simulink model "communication_Arduino"  (R2023b)
settings: Solver=VariableStepAuto  StartTime=0.0  StopTime=1  FixedStep=0.001  RelTol=1e-3  AbsTol=1e-3
undefined symbols (not defined in the file): g, LF, robot_conversions, robot_joints, X, Y, Z
libraries: sm_lib x13, nesl_utility x7, simulink_extras x6, cstblocks x6, instrumentseriallib x3, simulink x3
settings Model: Creator=ivano  LastModifiedBy=ivano
settings SolverCC: AlgebraicLoopSolver=TrustRegion  MaxZcPerStep=1
settings DataIOCC: LimitDataPoints=on  MaxDataPoints=10000  ReturnWorkspaceOutputs=off  ReturnWorkspaceOutputsName=data
settings OptimizationCC: DefaultParameterBehavior=Inlined  EnhancedBackFolding=on  PassReuseOutputArgsAs=Individual arguments  ZeroExternalMemoryAtStartup=off  ZeroInternalMemoryAtStartup=off  MaxStackSize=64  OptimizeBlockOrder=speed  DifferentSizesBufferReuse=on  OptimizationCustomize=off  EfficientTunableParamExpr=on
settings DebuggingCC: ParameterTunabilityLossMsg=error  UnconnectedInputMsg=warning  UnconnectedOutputMsg=warning  UnconnectedLineMsg=warning  AllowSymbolicDim=off  SubsystemReferenceDiagnosticForUnitTest=warning  SFUnexpectedBacktrackingDiag=warning  SFNoUnconditionalDefaultTransitionDiag=warning  SFExecutionAtInitializationDiag=none  ArithmeticOperatorsInVariantConditions=warning
settings HardwareCC: ProdBitPerPointer=32  ProdBitPerSizeT=32  ProdBitPerPtrDiffT=32  ProdLargestAtomicInteger=Long  ProdLargestAtomicFloat=Double  ProdWordSize=32  ProdHWDeviceType=ARM Compatible->ARM Cortex
settings ModelReferenceCC: EnableRefExpFcnMdlSchedulingChecks=on
settings SFSimCC: SimUseLocalCustomCode=off  MATLABDynamicMemAlloc=off  CustomCodeUndefinedFunction=UseInterfaceOnly  SimTargetLang=C++  GPUAcceleration=on  SimDLTargetLibrary=cudnn
settings RTWCC: Description=Embedded Coder  SystemTargetFile=ert.tlc  TemplateMakefile=ert_default_tmf  RTWUseLocalCustomCode=off  BuildConfiguration=Faster Runs  DLArmComputeVersion=19.05
settings CodeAppCC: ForceParamTrailComments=on  IgnoreCustomStorageClasses=off  OperatorAnnotations=on  SimulinkDataObjDesc=on  SFDataObjDesc=on  InsertBlockDesc=on
settings ERTTargetCC: SupportContinuousTime=on  ExtModeTransport=3  ExtModeStaticAlloc=on  ExtModeStaticAllocSize=24576  ExtModeMexFile=ext_xcp  ExtModeIntrfLevel=Level2 - Open  ERTCustomFileTemplate=example_file_process.tlc
settings ConfigComp: CovMetricSettings=dw  CovSaveCumulativeToWorkspaceVar=on  CovSaveSingleToWorkspaceVar=on  CovExternalEMLEnable=off  CovSFcnEnable=off
settings SimscapeCC: SimscapeLogType=all  SimscapeLogSimulationStatistics=on  SimscapeLogDataHistory=10000

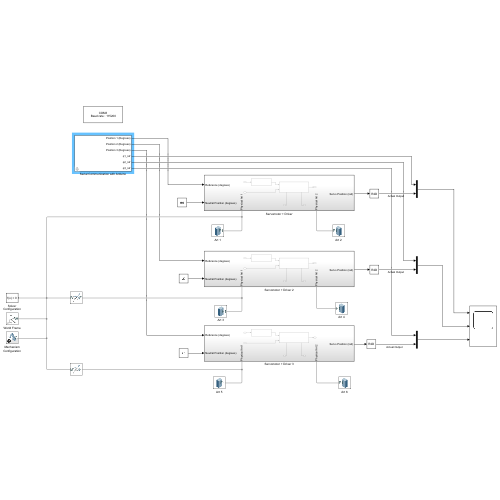
[thumbnail: Simulink's stored preview of the top-level diagram]
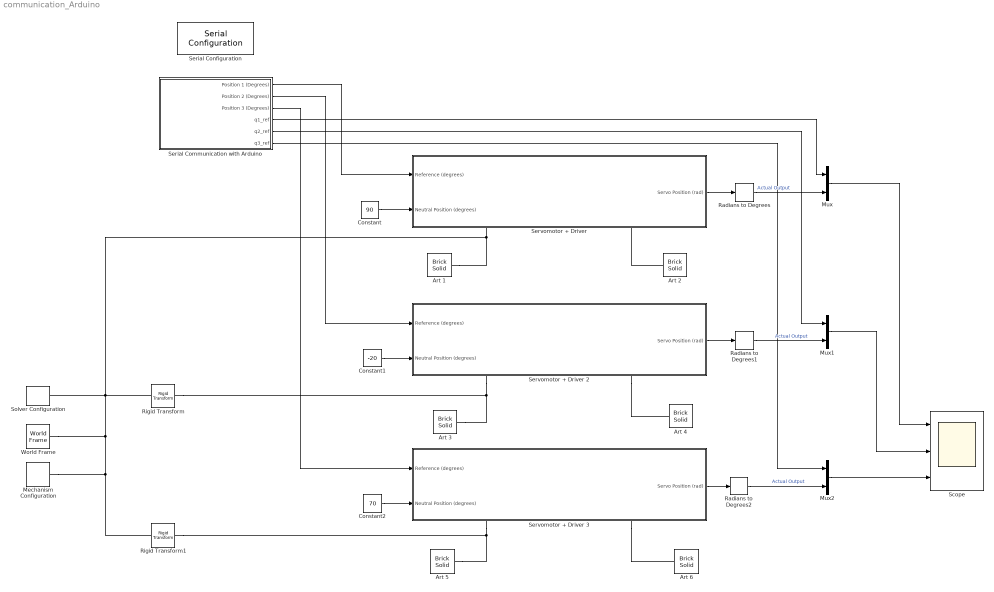
== system communication_Arduino ==
  Art 1 : sm_lib/Body Elements/Brick Solid  GraphicAmbientColor=[0.15 0.15 0.15 1.0]  BasedOnType=Density  BrickDimensions=[1 1 1]  BrickDimensionsUnits=m  CenterOfMass=[0 0 0]  CenterOfMassUnits=m  GraphicDiffuseColor=[0.0 0.8 0.8]  Density=10  DensityUnits=kg/m^3  DoExposeReferenceFrame=off  GraphicEmissiveColor=[0.0 0.0 0.0 1.0]  ExportEntireGeometry=off  SerializedFrames=<Frames><Frame><Id>Frame1</Id><Value><Name>F1</Name><Origin><Source>GeometricFeature</Source><FeatureName>+z surface</FeatureName></Origin><PrimaryAxis><DefinedDirection>+Z</DefinedDirection><Source>ReferenceFrame</Source><SourceDirection>+Z</SourceDirection><FeatureName></FeatureName></PrimaryAxis><SecondaryAxis><DefinedDirection>+X</DefinedDirection><Source>ReferenceFrame</Source><SourceDirection>+X</SourceDirection><FeatureName></FeatureName></SecondaryAxis></Value></Frame></Frames>  MarkerShape=Sphere  MarkerSize=10  GraphicType=FromGeometry  InertiaType=CalculateFromGeometry  Mass=1  MassUnits=kg  MomentsOfInertia=[1 1 1]  MomentsOfInertiaUnits=kg*m^2  GraphicOpacity=1.0  ProductsOfInertia=[0 0 0]  ProductsOfInertiaUnits=kg*m^2  GraphicShininess=75  GraphicSpecularColor=[0.5 0.5 0.5 1.0]  GraphicVisPropType=SimpleVisualProperties
  Art 2 : sm_lib/Body Elements/Brick Solid  GraphicAmbientColor=[0.15 0.15 0.15 1.0]  BasedOnType=Density  BrickDimensions=[3 1 1]  BrickDimensionsUnits=m  CenterOfMass=[0 0 0]  CenterOfMassUnits=m  GraphicDiffuseColor=[0.8 0.8 1.0]  Density=10  DensityUnits=kg/m^3  DoExposeReferenceFrame=off  GraphicEmissiveColor=[0.0 0.0 0.0 1.0]  ExportEntireGeometry=off  SerializedFrames=<Frames><Frame><Id>Frame1</Id><Value><Name>F1</Name><Origin><Source>GeometricFeature</Source><FeatureName>+z surface</FeatureName></Origin><PrimaryAxis><DefinedDirection>-Z</DefinedDirection><Source>ReferenceFrame</Source><SourceDirection>+Z</SourceDirection><FeatureName></FeatureName></PrimaryAxis><SecondaryAxis><DefinedDirection>+X</DefinedDirection><Source>ReferenceFrame</Source><SourceDirection>+X</SourceDirection><FeatureName></FeatureName></SecondaryAxis></Value></Frame></Frames>  MarkerShape=Sphere  MarkerSize=10  GraphicType=FromGeometry  InertiaType=CalculateFromGeometry  Mass=1  MassUnits=kg  MomentsOfInertia=[1 1 1]  MomentsOfInertiaUnits=kg*m^2  GraphicOpacity=1.0  ProductsOfInertia=[0 0 0]  ProductsOfInertiaUnits=kg*m^2  GraphicShininess=75  GraphicSpecularColor=[0.5 0.5 0.5 1.0]  GraphicVisPropType=SimpleVisualProperties
  Art 3 : sm_lib/Body Elements/Brick Solid  GraphicAmbientColor=[0.15 0.15 0.15 1.0]  BasedOnType=Density  BrickDimensions=[1 1 1]  BrickDimensionsUnits=m  CenterOfMass=[0 0 0]  CenterOfMassUnits=m  GraphicDiffuseColor=[0.0 0.8 0.8]  Density=10  DensityUnits=kg/m^3  DoExposeReferenceFrame=off  GraphicEmissiveColor=[0.0 0.0 0.0 1.0]  ExportEntireGeometry=off  SerializedFrames=<Frames><Frame><Id>Frame1</Id><Value><Name>F1</Name><Origin><Source>GeometricFeature</Source><FeatureName>+z surface</FeatureName></Origin><PrimaryAxis><DefinedDirection>+Z</DefinedDirection><Source>ReferenceFrame</Source><SourceDirection>+Z</SourceDirection><FeatureName></FeatureName></PrimaryAxis><SecondaryAxis><DefinedDirection>+X</DefinedDirection><Source>ReferenceFrame</Source><SourceDirection>+X</SourceDirection><FeatureName></FeatureName></SecondaryAxis></Value></Frame></Frames>  MarkerShape=Sphere  MarkerSize=10  GraphicType=FromGeometry  InertiaType=CalculateFromGeometry  Mass=1  MassUnits=kg  MomentsOfInertia=[1 1 1]  MomentsOfInertiaUnits=kg*m^2  GraphicOpacity=1.0  ProductsOfInertia=[0 0 0]  ProductsOfInertiaUnits=kg*m^2  GraphicShininess=75  GraphicSpecularColor=[0.5 0.5 0.5 1.0]  GraphicVisPropType=SimpleVisualProperties
  Art 4 : sm_lib/Body Elements/Brick Solid  GraphicAmbientColor=[0.15 0.15 0.15 1.0]  BasedOnType=Density  BrickDimensions=[3 1 1]  BrickDimensionsUnits=m  CenterOfMass=[0 0 0]  CenterOfMassUnits=m  GraphicDiffuseColor=[0.8 0.8 1.0]  Density=10  DensityUnits=kg/m^3  DoExposeReferenceFrame=off  GraphicEmissiveColor=[0.0 0.0 0.0 1.0]  ExportEntireGeometry=off  SerializedFrames=<Frames><Frame><Id>Frame1</Id><Value><Name>F1</Name><Origin><Source>GeometricFeature</Source><FeatureName>+z surface</FeatureName></Origin><PrimaryAxis><DefinedDirection>-Z</DefinedDirection><Source>ReferenceFrame</Source><SourceDirection>+Z</SourceDirection><FeatureName></FeatureName></PrimaryAxis><SecondaryAxis><DefinedDirection>+X</DefinedDirection><Source>ReferenceFrame</Source><SourceDirection>+X</SourceDirection><FeatureName></FeatureName></SecondaryAxis></Value></Frame></Frames>  MarkerShape=Sphere  MarkerSize=10  GraphicType=FromGeometry  InertiaType=CalculateFromGeometry  Mass=1  MassUnits=kg  MomentsOfInertia=[1 1 1]  MomentsOfInertiaUnits=kg*m^2  GraphicOpacity=1.0  ProductsOfInertia=[0 0 0]  ProductsOfInertiaUnits=kg*m^2  GraphicShininess=75  GraphicSpecularColor=[0.5 0.5 0.5 1.0]  GraphicVisPropType=SimpleVisualProperties
  Art 5 : sm_lib/Body Elements/Brick Solid  GraphicAmbientColor=[0.15 0.15 0.15 1.0]  BasedOnType=Density  BrickDimensions=[1 1 1]  BrickDimensionsUnits=m  CenterOfMass=[0 0 0]  CenterOfMassUnits=m  GraphicDiffuseColor=[0.0 0.8 0.8]  Density=10  DensityUnits=kg/m^3  DoExposeReferenceFrame=off  GraphicEmissiveColor=[0.0 0.0 0.0 1.0]  ExportEntireGeometry=off  SerializedFrames=<Frames><Frame><Id>Frame1</Id><Value><Name>F1</Name><Origin><Source>GeometricFeature</Source><FeatureName>+z surface</FeatureName></Origin><PrimaryAxis><DefinedDirection>+Z</DefinedDirection><Source>ReferenceFrame</Source><SourceDirection>+Z</SourceDirection><FeatureName></FeatureName></PrimaryAxis><SecondaryAxis><DefinedDirection>+X</DefinedDirection><Source>ReferenceFrame</Source><SourceDirection>+X</SourceDirection><FeatureName></FeatureName></SecondaryAxis></Value></Frame></Frames>  MarkerShape=Sphere  MarkerSize=10  GraphicType=FromGeometry  InertiaType=CalculateFromGeometry  Mass=1  MassUnits=kg  MomentsOfInertia=[1 1 1]  MomentsOfInertiaUnits=kg*m^2  GraphicOpacity=1.0  ProductsOfInertia=[0 0 0]  ProductsOfInertiaUnits=kg*m^2  GraphicShininess=75  GraphicSpecularColor=[0.5 0.5 0.5 1.0]  GraphicVisPropType=SimpleVisualProperties
  Art 6 : sm_lib/Body Elements/Brick Solid  GraphicAmbientColor=[0.15 0.15 0.15 1.0]  BasedOnType=Density  BrickDimensions=[3 1 1]  BrickDimensionsUnits=m  CenterOfMass=[0 0 0]  CenterOfMassUnits=m  GraphicDiffuseColor=[0.8 0.8 1.0]  Density=10  DensityUnits=kg/m^3  DoExposeReferenceFrame=off  GraphicEmissiveColor=[0.0 0.0 0.0 1.0]  ExportEntireGeometry=off  SerializedFrames=<Frames><Frame><Id>Frame1</Id><Value><Name>F1</Name><Origin><Source>GeometricFeature</Source><FeatureName>+z surface</FeatureName></Origin><PrimaryAxis><DefinedDirection>-Z</DefinedDirection><Source>ReferenceFrame</Source><SourceDirection>+Z</SourceDirection><FeatureName></FeatureName></PrimaryAxis><SecondaryAxis><DefinedDirection>+X</DefinedDirection><Source>ReferenceFrame</Source><SourceDirection>+X</SourceDirection><FeatureName></FeatureName></SecondaryAxis></Value></Frame></Frames>  MarkerShape=Sphere  MarkerSize=10  GraphicType=FromGeometry  InertiaType=CalculateFromGeometry  Mass=1  MassUnits=kg  MomentsOfInertia=[1 1 1]  MomentsOfInertiaUnits=kg*m^2  GraphicOpacity=1.0  ProductsOfInertia=[0 0 0]  ProductsOfInertiaUnits=kg*m^2  GraphicShininess=75  GraphicSpecularColor=[0.5 0.5 0.5 1.0]  GraphicVisPropType=SimpleVisualProperties
  Constant : Constant  Value=90
  Constant1 : Constant  Value=-20
  Constant2 : Constant  Value=70
  Mechanism Configuration : sm_lib/Utilities/Mechanism Configuration  UniformGravity=Constant  GravityVector=[0 0 g]  GravityVectorUnits=m/s^2  LinearizationDelta=0.001  JointModeTransitionNonlinearIterations=2
  Mux : Mux  Inputs=2
  Mux1 : Mux  Inputs=2
  Mux2 : Mux  Inputs=2
  Radians to Degrees : simulink_extras/Transformations/Radians to Degrees
  Radians to Degrees1 : simulink_extras/Transformations/Radians to Degrees
  Radians to Degrees2 : simulink_extras/Transformations/Radians to Degrees
  Rigid Transform : sm_lib/Frames and Transforms/Rigid Transform  TranslationMethod=Cartesian  TranslationStandardOffset=0  TranslationStandardOffsetUnits=m  TranslationStandardAxis=+Z  TranslationCartesianOffset=[5 0 0]  TranslationCartesianOffsetUnits=m  TranslationROffset=0  TranslationROffsetUnits=m  TranslationZOffset=0  TranslationZOffsetUnits=m  TranslationThetaOffset=0  TranslationThetaOffsetUnits=deg  RotationMethod=None  RotationAngleUnits=deg  RotationStandardAxis=+Z  RotationAngle=0.0  RotationArbitraryAxis=[0 0 1]  FollAlignAxisA=+X  BaseAlignAxisA=+Y  FollAlignAxisB=+Y  BaseAlignAxisB=+Z  RotationSequenceAxes=FollowerAxes  RotationSequence=XYX  RotationSequenceAngles=[0 0 0]  RotationSequenceAnglesUnits=deg  RotationMatrix=[1 0 0; 0 1 0; 0 0 1]  Quaternion=[1 0 0 0]
  Rigid Transform1 : sm_lib/Frames and Transforms/Rigid Transform  TranslationMethod=Cartesian  TranslationStandardOffset=0  TranslationStandardOffsetUnits=m  TranslationStandardAxis=+Z  TranslationCartesianOffset=[0 5 0]  TranslationCartesianOffsetUnits=m  TranslationROffset=0  TranslationROffsetUnits=m  TranslationZOffset=0  TranslationZOffsetUnits=m  TranslationThetaOffset=0  TranslationThetaOffsetUnits=deg  RotationMethod=None  RotationAngleUnits=deg  RotationStandardAxis=+Z  RotationAngle=0.0  RotationArbitraryAxis=[0 0 1]  FollAlignAxisA=+X  BaseAlignAxisA=+Y  FollAlignAxisB=+Y  BaseAlignAxisB=+Z  RotationSequenceAxes=FollowerAxes  RotationSequence=XYX  RotationSequenceAngles=[0 0 0]  RotationSequenceAnglesUnits=deg  RotationMatrix=[1 0 0; 0 1 0; 0 0 1]  Quaternion=[1 0 0 0]
  Scope : Scope  NumInputPorts=3
  Serial Communication with Arduino : Subsystem  mask{q1=0, q2=0, q3=0}
  Serial Configuration : instrumentseriallib/Serial Configuration  Priority=-200000  PortSel=COM3  Port=COM3  ComPort=COM3  BaudRate=115200  DataBits=8  Parity=none  StopBits=1  ByteOrder=little-endian  FlowControl=none  Timeout=10  SimulateUsing=Interpreted execution  BlockInModel=on  aMode=1
  Servomotor + Driver : Subsystem
      settings: PortSchema="{\"entries\":[{\"content\":{\"sides\":[{\"content\":{\"connectorIds\":[\"In1\",\"In2\"]},\"type\":\"ConnectorPlacement.EquallySpacedRectSide\",\"uuid\":\"34aed934-2639-4a00-aaee-cf3027466446\"},{\"content\":{\"connectorIds\":[\"Out1\"],\"side\":\"RIGHT\"},\"type\":\"ConnectorPlacement.EquallySpacedRectSide\",\"uuid\":\"6801890d-3466-4e37-90e8-6d1471e5b2c4\"},{\"content\":{\"side\":\"TOP\"},\"type\":\"ConnectorPlacement.EquallySpacedRectSide\",\"uuid\":\"bc3191aa-eca4-4e32-9fcf-8d5b7059b0b6\"},{\"content\":{\"connectorIds\":[\"RConn1\",\"RConn2\"],\"side\":\"BOTTOM\"},\"type\":\"ConnectorPlacement.EquallySpacedRectSide\",\"uuid\":\"867f09f9-bc2c-4353-bf05-5e7fc6d76fc7\"}]},\"type\":\"ConnectorPlacement.EquallySpacedConnector\",\"uuid\":\"7616468a-464c-41b8-bfd7-188201b948eb\"}],\"packageUris\":[\"http://schema.mathworks.com/mf0/Connector/R2020b\"],\"version\":\"1.0\"}"
  Servomotor + Driver 2 : Subsystem
      settings: PortSchema="{\"entries\":[{\"content\":{\"sides\":[{\"content\":{\"connectorIds\":[\"In1\",\"In2\"]},\"type\":\"ConnectorPlacement.EquallySpacedRectSide\",\"uuid\":\"34aed934-2639-4a00-aaee-cf3027466446\"},{\"content\":{\"connectorIds\":[\"Out1\"],\"side\":\"RIGHT\"},\"type\":\"ConnectorPlacement.EquallySpacedRectSide\",\"uuid\":\"6801890d-3466-4e37-90e8-6d1471e5b2c4\"},{\"content\":{\"side\":\"TOP\"},\"type\":\"ConnectorPlacement.EquallySpacedRectSide\",\"uuid\":\"bc3191aa-eca4-4e32-9fcf-8d5b7059b0b6\"},{\"content\":{\"connectorIds\":[\"RConn1\",\"RConn2\"],\"side\":\"BOTTOM\"},\"type\":\"ConnectorPlacement.EquallySpacedRectSide\",\"uuid\":\"867f09f9-bc2c-4353-bf05-5e7fc6d76fc7\"}]},\"type\":\"ConnectorPlacement.EquallySpacedConnector\",\"uuid\":\"7616468a-464c-41b8-bfd7-188201b948eb\"}],\"packageUris\":[\"http://schema.mathworks.com/mf0/Connector/R2020b\"],\"version\":\"1.0\"}"
  Servomotor + Driver 3 : Subsystem
      settings: PortSchema="{\"entries\":[{\"content\":{\"sides\":[{\"content\":{\"connectorIds\":[\"In1\",\"In2\"]},\"type\":\"ConnectorPlacement.EquallySpacedRectSide\",\"uuid\":\"34aed934-2639-4a00-aaee-cf3027466446\"},{\"content\":{\"connectorIds\":[\"Out1\"],\"side\":\"RIGHT\"},\"type\":\"ConnectorPlacement.EquallySpacedRectSide\",\"uuid\":\"6801890d-3466-4e37-90e8-6d1471e5b2c4\"},{\"content\":{\"side\":\"TOP\"},\"type\":\"ConnectorPlacement.EquallySpacedRectSide\",\"uuid\":\"bc3191aa-eca4-4e32-9fcf-8d5b7059b0b6\"},{\"content\":{\"connectorIds\":[\"RConn1\",\"RConn2\"],\"side\":\"BOTTOM\"},\"type\":\"ConnectorPlacement.EquallySpacedRectSide\",\"uuid\":\"867f09f9-bc2c-4353-bf05-5e7fc6d76fc7\"}]},\"type\":\"ConnectorPlacement.EquallySpacedConnector\",\"uuid\":\"7616468a-464c-41b8-bfd7-188201b948eb\"}],\"packageUris\":[\"http://schema.mathworks.com/mf0/Connector/R2020b\"],\"version\":\"1.0\"}"
  Solver Configuration : nesl_utility/Solver Configuration  PhysicalDomain=network_engine_domain  SubClassName=solver  LeftPortType=input  RightPortType=generic  Tones=[]  Harmonics=[]  SimulateNoise=off  Profile=off  UseLocalSampling=off  EnableSwitchedLinearOptims=on  FrequencyDomain=off  UseCCode=off  RelTol=0.001  AbsTol=1e-06  MinStep=1e-09  ToWorkspace=off  RevertToSquareIcSolve=off  NumHomotopyIterations=100  PhasorMode=off  PhasorModeNumHarmonics=1  ConsistencySolver=NEWTON_XTOL_AFTER_FTOL  IndexReductionMethod=DerivativeReplacement  DoDC=off  ResidualTolerance=1e-09  ConsistencyTolSource=GLOBAL  ConsistencyAbsTol=0.001  ConsistencyRelTol=0.001  ConsistencyTolFactor=0.001  UseLocalSolver=off  LocalSolverChoice=NE_BACKWARD_EULER_ADVANCER  ResolveIndetEquations=on  FunctionEvalNumThread=1  LocalSolverSampleTime=0.001  DoFixedCost=off  MaxNonlinIter=3  MaxModeIter=2  ComputeImpulses=off  ImpulseIterations=2  LinearAlgebra=Sparse  LinearAlgebraNumThread=0  EquationFormulation=NE_TIME_EF  DelaysMemoryBudget=1024  AutomaticFiltering=on  FilteringTimeConstant=0.001  PartitionStorageMethod=AS_NEEDED  PartitionMemoryBudget=1024  PartitionMethod=FAST  MultibodyUseLocalSolver=off  MultibodyLocalSolverChoice=ODE1  MultibodyLocalSolverSampleTime=0.001
  World Frame : sm_lib/Frames and Transforms/World Frame
  wires:
  Radians to Degrees/1 -> Mux/2  "Actual Output"
  Mux/1 -> Scope/1
  Servomotor + Driver/1(Servo Position (rad)) -> Radians to Degrees/1
  Radians to Degrees1/1 -> Mux1/2  "Actual Output"
  Mux1/1 -> Scope/2
  Servomotor + Driver 2/1(Servo Position (rad)) -> Radians to Degrees1/1
  Radians to Degrees2/1 -> Mux2/2  "Actual Output"
  Mux2/1 -> Scope/3
  Servomotor + Driver 3/1(Servo Position (rad)) -> Radians to Degrees2/1
  Serial Communication with Arduino/4(q1_ref) -> Mux/1
  Serial Communication with Arduino/5(q2_ref) -> Mux1/1
  Serial Communication with Arduino/6(q3_ref) -> Mux2/1
  Serial Communication with Arduino/1(Position 1 (Degrees)) -> Servomotor + Driver/1(Reference (degrees))
  Serial Communication with Arduino/2(Position 2 (Degrees)) -> Servomotor + Driver 2/1(Reference (degrees))
  Serial Communication with Arduino/3(Position 3 (Degrees)) -> Servomotor + Driver 3/1(Reference (degrees))
  Constant/1 -> Servomotor + Driver/2(Neutral Position (degrees))
  Constant1/1 -> Servomotor + Driver 2/2(Neutral Position (degrees))
  Constant2/1 -> Servomotor + Driver 3/2(Neutral Position (degrees))
  connections:
  World Frame/RConn1 -- Rigid Transform/LConn1 -- Art 1/LConn1 -- Servomotor + Driver/RConn1 -- Solver Configuration/RConn1 -- Mechanism Configuration/RConn1 -- Rigid Transform1/LConn1
  Art 2/LConn1 -- Servomotor + Driver/RConn2
  Art 3/LConn1 -- Servomotor + Driver 2/RConn1 -- Rigid Transform/RConn1
  Servomotor + Driver 2/RConn2 -- Art 4/LConn1
  Art 5/LConn1 -- Servomotor + Driver 3/RConn1 -- Rigid Transform1/RConn1
  Servomotor + Driver 3/RConn2 -- Art 6/LConn1

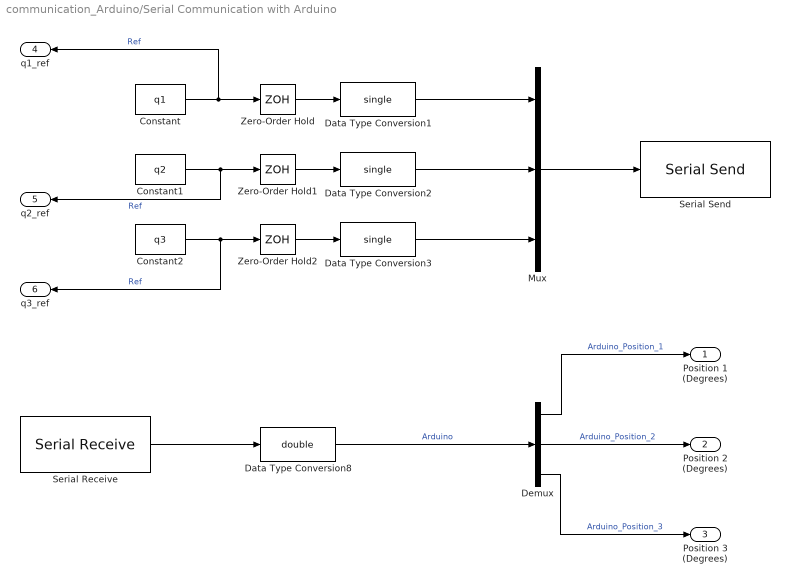
== system communication_Arduino/Serial Communication with Arduino ==
  Constant : Constant  Value=q1
  Constant1 : Constant  Value=q2
  Constant2 : Constant  Value=q3
  Data Type Conversion1 : DataTypeConversion  OutDataTypeStr=single  SaturateOnIntegerOverflow=off  RndMeth=Floor
  Data Type Conversion2 : DataTypeConversion  OutDataTypeStr=single  SaturateOnIntegerOverflow=off  RndMeth=Floor
  Data Type Conversion3 : DataTypeConversion  OutDataTypeStr=single  SaturateOnIntegerOverflow=off  RndMeth=Floor
  Data Type Conversion8 : DataTypeConversion  OutDataTypeStr=double  SaturateOnIntegerOverflow=off  RndMeth=Floor
  Demux : Demux  Outputs=3
  Mux : Mux  Inputs=3
  Serial Receive : instrumentseriallib/Serial Receive  Priority=1  PortSel=COM3  Port=COM3  ComPort=COM3  DataType=single  SaveDataType=uint8  ToggleHeader=on  Header='S'  DataSize=[3 1]  ToggleTerminator=on  Terminator=LF ('\n')  CustomTerminator=[]  InputFormat=Column major  ToggleDataSize=on  EnableBlockingMode=on  ActionDataUnavailable=Output last received value  ActionWhenDataUnavailable=Output last received value  CustomValue=0  SampleTime=0.01  SimulateUsing=Interpreted execution  BlockInModel=on  aMode=1
  Serial Send : instrumentseriallib/Serial Send  Priority=1  PortSel=COM3  Port=COM3  ComPort=COM3  Header='A'  Terminator=LF ('\n')  CustomTerminator=[]  EnableBlockingMode=on  SimulateUsing=Interpreted execution  BlockInModel=on  aMode=1
  Zero-Order Hold : ZeroOrderHold  SampleTime=0.01
  Zero-Order Hold1 : ZeroOrderHold  SampleTime=0.01
  Zero-Order Hold2 : ZeroOrderHold  SampleTime=0.01
  Position 1 (Degrees) : Outport
  Position 2 (Degrees) : Outport  Port=2
  Position 3 (Degrees) : Outport  Port=3
  q1_ref : Outport  Port=4
  q2_ref : Outport  Port=5
  q3_ref : Outport  Port=6
  wires:
  Constant/1 -> q1_ref/1, Zero-Order Hold/1  "Ref"
  Zero-Order Hold/1 -> Data Type Conversion1/1
  Constant1/1 -> q2_ref/1, Zero-Order Hold1/1  "Ref"
  Zero-Order Hold1/1 -> Data Type Conversion2/1
  Constant2/1 -> q3_ref/1, Zero-Order Hold2/1  "Ref"
  Zero-Order Hold2/1 -> Data Type Conversion3/1
  Data Type Conversion1/1 -> Mux/1
  Data Type Conversion2/1 -> Mux/2
  Data Type Conversion3/1 -> Mux/3
  Mux/1 -> Serial Send/1
  Demux/1 -> Position 1 (Degrees)/1  "Arduino_Position_1"
  Demux/2 -> Position 2 (Degrees)/1  "Arduino_Position_2"
  Demux/3 -> Position 3 (Degrees)/1  "Arduino_Position_3"
  Serial Receive/1 -> Data Type Conversion8/1
  Data Type Conversion8/1 -> Demux/1  "Arduino"

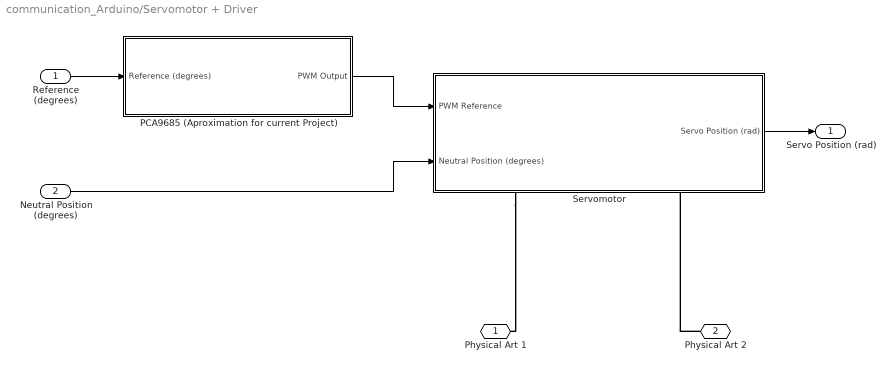
== system communication_Arduino/Servomotor + Driver ==
  Reference (degrees) : Inport
  Neutral Position (degrees) : Inport  Port=2
  PCA9685 (Aproximation for current Project) : Subsystem
  Servomotor : Subsystem
      settings: PortSchema="{\"entries\":[{\"content\":{\"sides\":[{\"content\":{\"connectorIds\":[\"In1\",\"In2\"]},\"type\":\"ConnectorPlacement.EquallySpacedRectSide\",\"uuid\":\"eeff66d3-7cb0-4fe9-90b5-92935711e170\"},{\"content\":{\"connectorIds\":[\"Out1\"],\"side\":\"RIGHT\"},\"type\":\"ConnectorPlacement.EquallySpacedRectSide\",\"uuid\":\"4c1729b3-3224-4ed4-9eed-359312bd5e7e\"},{\"content\":{\"side\":\"TOP\"},\"type\":\"ConnectorPlacement.EquallySpacedRectSide\",\"uuid\":\"ee6ed6e9-0c82-482d-bf53-5898b89012ab\"},{\"content\":{\"connectorIds\":[\"RConn1\",\"RConn2\"],\"side\":\"BOTTOM\"},\"type\":\"ConnectorPlacement.EquallySpacedRectSide\",\"uuid\":\"6da00c0c-ced6-4450-8de1-d587d7c692e9\"}]},\"type\":\"ConnectorPlacement.EquallySpacedConnector\",\"uuid\":\"38b9234f-cec7-4245-8a78-4426dc0791bf\"}],\"packageUris\":[\"http://schema.mathworks.com/mf0/Connector/R2020b\"],\"version\":\"1.0\"}"
  Physical Art 1 : PMIOPort  Side=Right
  Physical Art 2 : PMIOPort  Port=2  Side=Right
  Servo Position (rad) : Outport
  wires:
  PCA9685 (Aproximation for current Project)/1(PWM Output) -> Servomotor/1(PWM Reference)
  Neutral Position (degrees)/1 -> Servomotor/2(Neutral Position (degrees))
  Reference (degrees)/1 -> PCA9685 (Aproximation for current Project)/1(Reference (degrees))
  Servomotor/1(Servo Position (rad)) -> Servo Position (rad)/1
  connections:
  Servomotor/RConn1 -- Physical Art 1/RConn1
  Physical Art 2/RConn1 -- Servomotor/RConn2

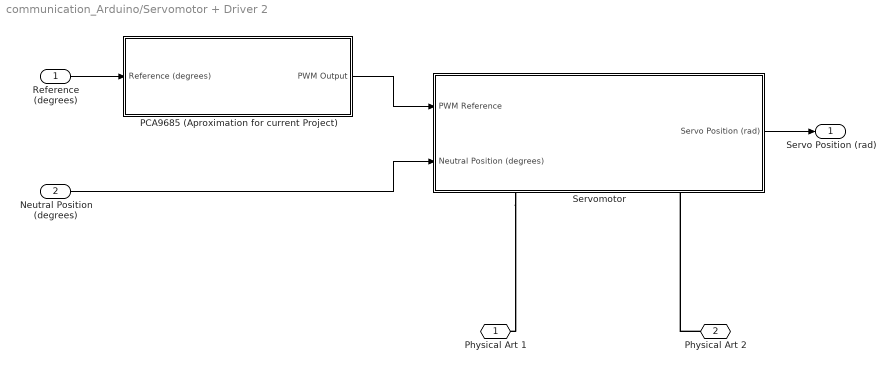
== system communication_Arduino/Servomotor + Driver 2 ==
  Reference (degrees) : Inport
  Neutral Position (degrees) : Inport  Port=2
  PCA9685 (Aproximation for current Project) : Subsystem
  Servomotor : Subsystem
      settings: PortSchema="{\"entries\":[{\"content\":{\"sides\":[{\"content\":{\"connectorIds\":[\"In1\",\"In2\"]},\"type\":\"ConnectorPlacement.EquallySpacedRectSide\",\"uuid\":\"eeff66d3-7cb0-4fe9-90b5-92935711e170\"},{\"content\":{\"connectorIds\":[\"Out1\"],\"side\":\"RIGHT\"},\"type\":\"ConnectorPlacement.EquallySpacedRectSide\",\"uuid\":\"4c1729b3-3224-4ed4-9eed-359312bd5e7e\"},{\"content\":{\"side\":\"TOP\"},\"type\":\"ConnectorPlacement.EquallySpacedRectSide\",\"uuid\":\"ee6ed6e9-0c82-482d-bf53-5898b89012ab\"},{\"content\":{\"connectorIds\":[\"RConn1\",\"RConn2\"],\"side\":\"BOTTOM\"},\"type\":\"ConnectorPlacement.EquallySpacedRectSide\",\"uuid\":\"6da00c0c-ced6-4450-8de1-d587d7c692e9\"}]},\"type\":\"ConnectorPlacement.EquallySpacedConnector\",\"uuid\":\"38b9234f-cec7-4245-8a78-4426dc0791bf\"}],\"packageUris\":[\"http://schema.mathworks.com/mf0/Connector/R2020b\"],\"version\":\"1.0\"}"
  Physical Art 1 : PMIOPort  Side=Right
  Physical Art 2 : PMIOPort  Port=2  Side=Right
  Servo Position (rad) : Outport
  wires:
  PCA9685 (Aproximation for current Project)/1(PWM Output) -> Servomotor/1(PWM Reference)
  Neutral Position (degrees)/1 -> Servomotor/2(Neutral Position (degrees))
  Reference (degrees)/1 -> PCA9685 (Aproximation for current Project)/1(Reference (degrees))
  Servomotor/1(Servo Position (rad)) -> Servo Position (rad)/1
  connections:
  Servomotor/RConn1 -- Physical Art 1/RConn1
  Physical Art 2/RConn1 -- Servomotor/RConn2

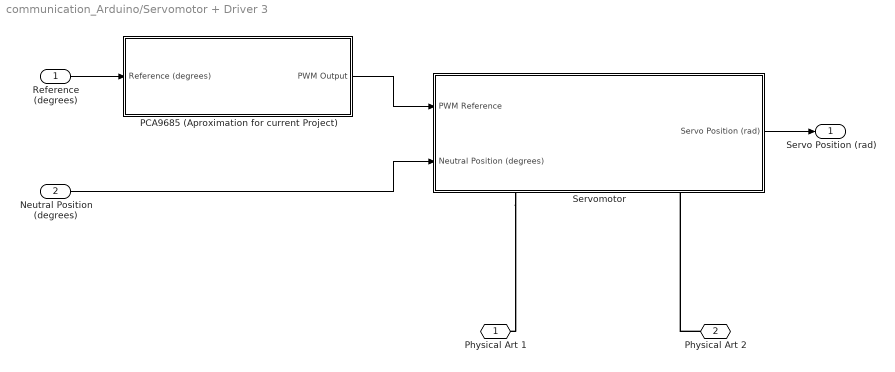
== system communication_Arduino/Servomotor + Driver 3 ==
  Reference (degrees) : Inport
  Neutral Position (degrees) : Inport  Port=2
  PCA9685 (Aproximation for current Project) : Subsystem
  Servomotor : Subsystem
      settings: PortSchema="{\"entries\":[{\"content\":{\"sides\":[{\"content\":{\"connectorIds\":[\"In1\",\"In2\"]},\"type\":\"ConnectorPlacement.EquallySpacedRectSide\",\"uuid\":\"eeff66d3-7cb0-4fe9-90b5-92935711e170\"},{\"content\":{\"connectorIds\":[\"Out1\"],\"side\":\"RIGHT\"},\"type\":\"ConnectorPlacement.EquallySpacedRectSide\",\"uuid\":\"4c1729b3-3224-4ed4-9eed-359312bd5e7e\"},{\"content\":{\"side\":\"TOP\"},\"type\":\"ConnectorPlacement.EquallySpacedRectSide\",\"uuid\":\"ee6ed6e9-0c82-482d-bf53-5898b89012ab\"},{\"content\":{\"connectorIds\":[\"RConn1\",\"RConn2\"],\"side\":\"BOTTOM\"},\"type\":\"ConnectorPlacement.EquallySpacedRectSide\",\"uuid\":\"6da00c0c-ced6-4450-8de1-d587d7c692e9\"}]},\"type\":\"ConnectorPlacement.EquallySpacedConnector\",\"uuid\":\"38b9234f-cec7-4245-8a78-4426dc0791bf\"}],\"packageUris\":[\"http://schema.mathworks.com/mf0/Connector/R2020b\"],\"version\":\"1.0\"}"
  Physical Art 1 : PMIOPort  Side=Right
  Physical Art 2 : PMIOPort  Port=2  Side=Right
  Servo Position (rad) : Outport
  wires:
  PCA9685 (Aproximation for current Project)/1(PWM Output) -> Servomotor/1(PWM Reference)
  Neutral Position (degrees)/1 -> Servomotor/2(Neutral Position (degrees))
  Reference (degrees)/1 -> PCA9685 (Aproximation for current Project)/1(Reference (degrees))
  Servomotor/1(Servo Position (rad)) -> Servo Position (rad)/1
  connections:
  Servomotor/RConn1 -- Physical Art 1/RConn1
  Physical Art 2/RConn1 -- Servomotor/RConn2

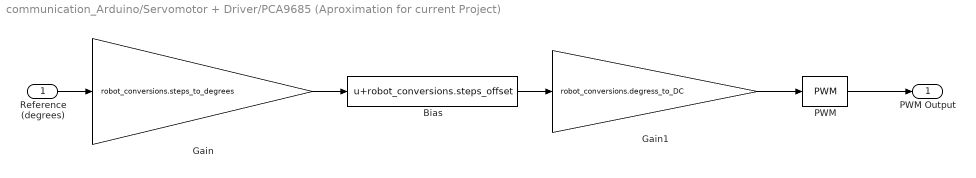
== system communication_Arduino/Servomotor + Driver/PCA9685 (Aproximation for current Project) ==
  Reference (degrees) : Inport
  Bias : Bias  Bias=robot_conversions.steps_offset  SaturateOnIntegerOverflow=off
  Gain : Gain  Gain=robot_conversions.steps_to_degrees
  Gain1 : Gain  Gain=robot_conversions.degress_to_DC
  PWM : simulink/Discontinuities/PWM  DisableCoverage=on  Period=0.02  InitialDelay=0  DisallowZeroDutyCycle=off  RunAtFixedTimeIntervals=off  SampleTime=0.01
  PWM Output : Outport
  wires:
  Gain/1 -> Bias/1
  Bias/1 -> Gain1/1
  Gain1/1 -> PWM/1
  Reference (degrees)/1 -> Gain/1
  PWM/1 -> PWM Output/1

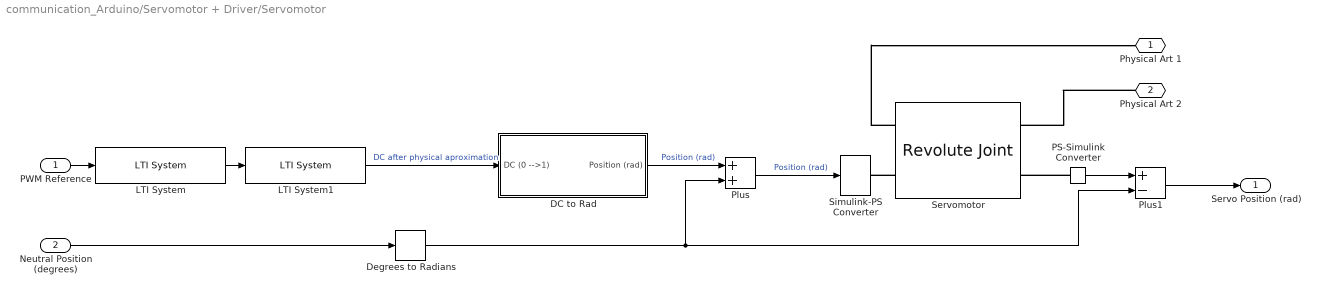
== system communication_Arduino/Servomotor + Driver/Servomotor ==
  PWM Reference : Inport
  Neutral Position (degrees) : Inport  Port=2
  DC to Rad : Subsystem
  Degrees to Radians : simulink_extras/Transformations/Degrees to Radians
  LTI System : cstblocks/LTI System  sys=robot_tf.bessel_filter  IC=[]  PadeOrder=0
  LTI System1 : cstblocks/LTI System  sys=robot_tf.physical_tf  IC=[]  PadeOrder=0
  PS-Simulink Converter : nesl_utility/PS-Simulink Converter  PhysicalDomain=network_engine_domain  SubClassName=ps_output  LeftPortType=input  RightPortType=output  PseudoPeriodic=off  Frequencies=[]  VectorFormat=inherit  Unit=inherit  AffineConversion=off
  Plus : Sum
  Plus1 : Sum  Inputs=+-
  Servomotor : sm_lib/Joints/Revolute Joint  JointMode=Normal  SenseConstraintForce=off  SenseConstraintForceX=off  SenseConstraintForceY=off  SenseConstraintForceZ=off  SenseConstraintTorque=off  SenseConstraintTorqueX=off  SenseConstraintTorqueY=off  SenseConstraintTorqueZ=off  SenseTotalForce=off  SenseTotalForceX=off  SenseTotalForceY=off  SenseTotalForceZ=off  SenseTotalTorque=off  SenseTotalTorqueX=off  SenseTotalTorqueY=off  SenseTotalTorqueZ=off  CompositeWrenchDir=FollowerOnBase  CompositeWrenchFrame=BaseFrame  EquilibriumPosition=0  EquilibriumPositionUnits=rad  SpringStiffness=0  SpringStiffnessUnits=N*m/deg  DampingCoefficient=0  DampingCoefficientUnits=N*m/(deg/s)  TorqueActuationMode=ComputedTorque  MotionActuationMode=InputMotion  SensePosition=on  SenseVelocity=off  SenseAcceleration=off  SenseTorqueForce=off  SenseLowerLimitTorqueForce=off  SenseUpperLimitTorqueForce=off  LowerLimitSpecify=on  LowerLimitBound=robot_joints.q_limits(1)  LowerLimitBoundUnits=rad  LowerLimitStiffness=1e4  LowerLimitStiffnessUnits=N*m/deg  LowerLimitDamping=10  LowerLimitDampingUnits=N*m/(deg/s)  LowerLimitTransitionRegionWidth=0.1  LowerLimitTransitionRegionWidthUnits=deg  UpperLimitSpecify=on  UpperLimitBound=robot_joints.q_limits(2)  UpperLimitBoundUnits=rad  UpperLimitStiffness=1e4  UpperLimitStiffnessUnits=N*m/deg  UpperLimitDamping=10  UpperLimitDampingUnits=N*m/(deg/s)  UpperLimitTransitionRegionWidth=0.1  UpperLimitTransitionRegionWidthUnits=deg  PositionTargetSpecify=off  PositionTargetPriority=High  PositionTargetValue=0  PositionTargetValueUnits=deg  VelocityTargetSpecify=off  VelocityTargetPriority=High  VelocityTargetValue=0  VelocityTargetValueUnits=deg/s
  Simulink-PS Converter : nesl_utility/Simulink-PS Converter  PhysicalDomain=network_engine_domain  SubClassName=ps_input  LeftPortType=input  RightPortType=output  PseudoPeriodic=off  Frequencies=[]  NoiseDistribution=none  NoiseParameters=[]  Unit=1  AffineConversion=off  FilteringAndDerivatives=filter  SimscapeFilterOrder=2  InputFilterTimeConstant=0.001  UdotUserProvided=0
  Physical Art 1 : PMIOPort  Side=Right
  Physical Art 2 : PMIOPort  Port=2  Side=Right
  Servo Position (rad) : Outport
  wires:
  PWM Reference/1 -> LTI System/1
  LTI System/1 -> LTI System1/1
  LTI System1/1 -> DC to Rad/1(DC (0 -->1))  "DC after physical aproximation"
  Neutral Position (degrees)/1 -> Degrees to Radians/1
  DC to Rad/1(Position (rad)) -> Plus/1  "Position (rad)"
  Plus/1 -> Simulink-PS Converter/1  "Position (rad)"
  Degrees to Radians/1 -> Plus1/2, Plus/2
  PS-Simulink Converter/1 -> Plus1/1
  Plus1/1 -> Servo Position (rad)/1
  connections:
  PS-Simulink Converter/LConn1 -- Servomotor/RConn2
  Physical Art 2/RConn1 -- Servomotor/RConn1
  Servomotor/LConn1 -- Physical Art 1/RConn1
  Servomotor/LConn2 -- Simulink-PS Converter/RConn1

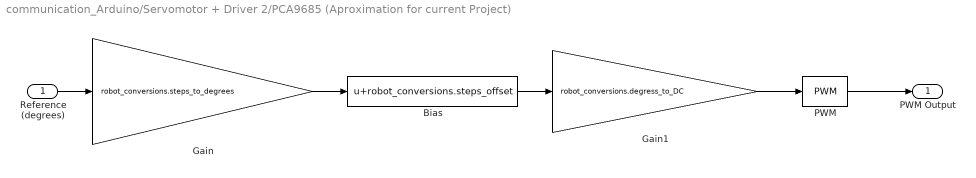
== system communication_Arduino/Servomotor + Driver 2/PCA9685 (Aproximation for current Project) ==
  Reference (degrees) : Inport
  Bias : Bias  Bias=robot_conversions.steps_offset  SaturateOnIntegerOverflow=off
  Gain : Gain  Gain=robot_conversions.steps_to_degrees
  Gain1 : Gain  Gain=robot_conversions.degress_to_DC
  PWM : simulink/Discontinuities/PWM  DisableCoverage=on  Period=0.02  InitialDelay=0  DisallowZeroDutyCycle=off  RunAtFixedTimeIntervals=off  SampleTime=0.01
  PWM Output : Outport
  wires:
  Gain/1 -> Bias/1
  Bias/1 -> Gain1/1
  Gain1/1 -> PWM/1
  Reference (degrees)/1 -> Gain/1
  PWM/1 -> PWM Output/1

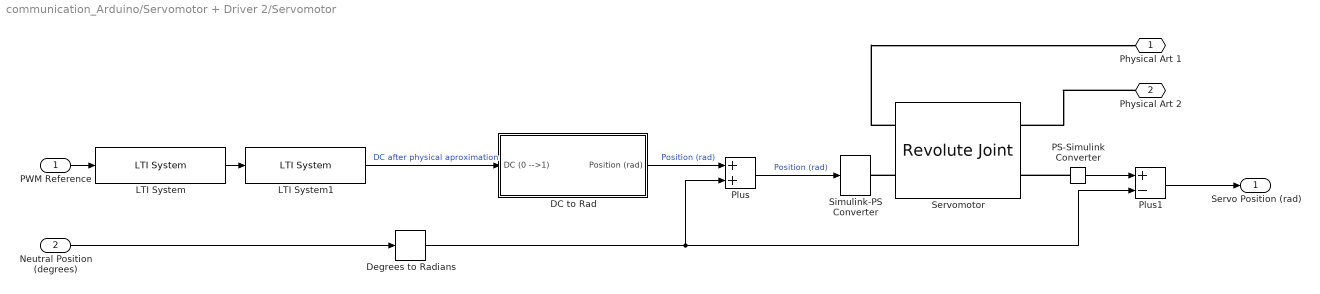
== system communication_Arduino/Servomotor + Driver 2/Servomotor ==
  PWM Reference : Inport
  Neutral Position (degrees) : Inport  Port=2
  DC to Rad : Subsystem
  Degrees to Radians : simulink_extras/Transformations/Degrees to Radians
  LTI System : cstblocks/LTI System  sys=robot_tf.bessel_filter  IC=[]  PadeOrder=0
  LTI System1 : cstblocks/LTI System  sys=robot_tf.physical_tf  IC=[]  PadeOrder=0
  PS-Simulink Converter : nesl_utility/PS-Simulink Converter  PhysicalDomain=network_engine_domain  SubClassName=ps_output  LeftPortType=input  RightPortType=output  PseudoPeriodic=off  Frequencies=[]  VectorFormat=inherit  Unit=inherit  AffineConversion=off
  Plus : Sum
  Plus1 : Sum  Inputs=+-
  Servomotor : sm_lib/Joints/Revolute Joint  JointMode=Normal  SenseConstraintForce=off  SenseConstraintForceX=off  SenseConstraintForceY=off  SenseConstraintForceZ=off  SenseConstraintTorque=off  SenseConstraintTorqueX=off  SenseConstraintTorqueY=off  SenseConstraintTorqueZ=off  SenseTotalForce=off  SenseTotalForceX=off  SenseTotalForceY=off  SenseTotalForceZ=off  SenseTotalTorque=off  SenseTotalTorqueX=off  SenseTotalTorqueY=off  SenseTotalTorqueZ=off  CompositeWrenchDir=FollowerOnBase  CompositeWrenchFrame=BaseFrame  EquilibriumPosition=0  EquilibriumPositionUnits=rad  SpringStiffness=0  SpringStiffnessUnits=N*m/deg  DampingCoefficient=0  DampingCoefficientUnits=N*m/(deg/s)  TorqueActuationMode=ComputedTorque  MotionActuationMode=InputMotion  SensePosition=on  SenseVelocity=off  SenseAcceleration=off  SenseTorqueForce=off  SenseLowerLimitTorqueForce=off  SenseUpperLimitTorqueForce=off  LowerLimitSpecify=on  LowerLimitBound=robot_joints.q_limits(1)  LowerLimitBoundUnits=rad  LowerLimitStiffness=1e4  LowerLimitStiffnessUnits=N*m/deg  LowerLimitDamping=10  LowerLimitDampingUnits=N*m/(deg/s)  LowerLimitTransitionRegionWidth=0.1  LowerLimitTransitionRegionWidthUnits=deg  UpperLimitSpecify=on  UpperLimitBound=robot_joints.q_limits(2)  UpperLimitBoundUnits=rad  UpperLimitStiffness=1e4  UpperLimitStiffnessUnits=N*m/deg  UpperLimitDamping=10  UpperLimitDampingUnits=N*m/(deg/s)  UpperLimitTransitionRegionWidth=0.1  UpperLimitTransitionRegionWidthUnits=deg  PositionTargetSpecify=off  PositionTargetPriority=High  PositionTargetValue=0  PositionTargetValueUnits=deg  VelocityTargetSpecify=off  VelocityTargetPriority=High  VelocityTargetValue=0  VelocityTargetValueUnits=deg/s
  Simulink-PS Converter : nesl_utility/Simulink-PS Converter  PhysicalDomain=network_engine_domain  SubClassName=ps_input  LeftPortType=input  RightPortType=output  PseudoPeriodic=off  Frequencies=[]  NoiseDistribution=none  NoiseParameters=[]  Unit=1  AffineConversion=off  FilteringAndDerivatives=filter  SimscapeFilterOrder=2  InputFilterTimeConstant=0.001  UdotUserProvided=0
  Physical Art 1 : PMIOPort  Side=Right
  Physical Art 2 : PMIOPort  Port=2  Side=Right
  Servo Position (rad) : Outport
  wires:
  PWM Reference/1 -> LTI System/1
  LTI System/1 -> LTI System1/1
  LTI System1/1 -> DC to Rad/1(DC (0 -->1))  "DC after physical aproximation"
  Neutral Position (degrees)/1 -> Degrees to Radians/1
  DC to Rad/1(Position (rad)) -> Plus/1  "Position (rad)"
  Plus/1 -> Simulink-PS Converter/1  "Position (rad)"
  Degrees to Radians/1 -> Plus1/2, Plus/2
  PS-Simulink Converter/1 -> Plus1/1
  Plus1/1 -> Servo Position (rad)/1
  connections:
  PS-Simulink Converter/LConn1 -- Servomotor/RConn2
  Physical Art 2/RConn1 -- Servomotor/RConn1
  Servomotor/LConn1 -- Physical Art 1/RConn1
  Servomotor/LConn2 -- Simulink-PS Converter/RConn1

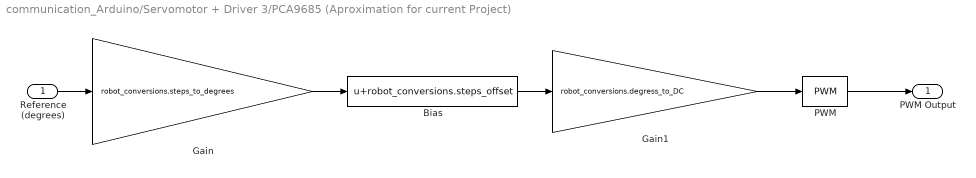
== system communication_Arduino/Servomotor + Driver 3/PCA9685 (Aproximation for current Project) ==
  Reference (degrees) : Inport
  Bias : Bias  Bias=robot_conversions.steps_offset  SaturateOnIntegerOverflow=off
  Gain : Gain  Gain=robot_conversions.steps_to_degrees
  Gain1 : Gain  Gain=robot_conversions.degress_to_DC
  PWM : simulink/Discontinuities/PWM  DisableCoverage=on  Period=0.02  InitialDelay=0  DisallowZeroDutyCycle=off  RunAtFixedTimeIntervals=off  SampleTime=0.01
  PWM Output : Outport
  wires:
  Gain/1 -> Bias/1
  Bias/1 -> Gain1/1
  Gain1/1 -> PWM/1
  Reference (degrees)/1 -> Gain/1
  PWM/1 -> PWM Output/1

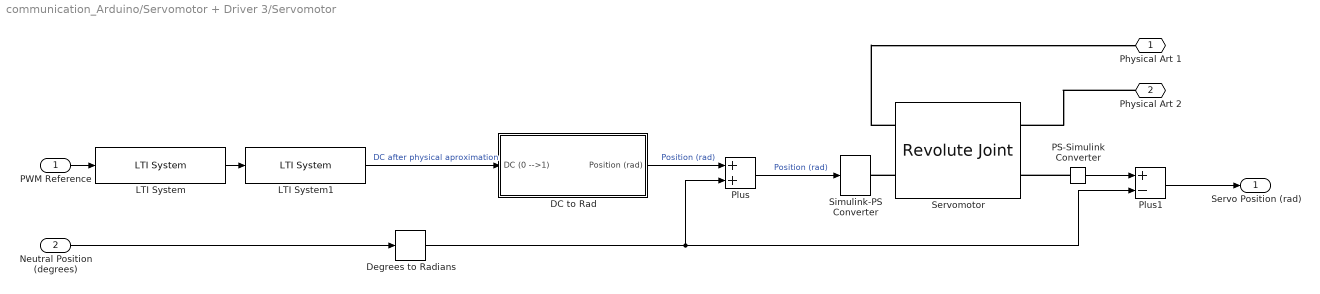
== system communication_Arduino/Servomotor + Driver 3/Servomotor ==
  PWM Reference : Inport
  Neutral Position (degrees) : Inport  Port=2
  DC to Rad : Subsystem
  Degrees to Radians : simulink_extras/Transformations/Degrees to Radians
  LTI System : cstblocks/LTI System  sys=robot_tf.bessel_filter  IC=[]  PadeOrder=0
  LTI System1 : cstblocks/LTI System  sys=robot_tf.physical_tf  IC=[]  PadeOrder=0
  PS-Simulink Converter : nesl_utility/PS-Simulink Converter  PhysicalDomain=network_engine_domain  SubClassName=ps_output  LeftPortType=input  RightPortType=output  PseudoPeriodic=off  Frequencies=[]  VectorFormat=inherit  Unit=inherit  AffineConversion=off
  Plus : Sum
  Plus1 : Sum  Inputs=+-
  Servomotor : sm_lib/Joints/Revolute Joint  JointMode=Normal  SenseConstraintForce=off  SenseConstraintForceX=off  SenseConstraintForceY=off  SenseConstraintForceZ=off  SenseConstraintTorque=off  SenseConstraintTorqueX=off  SenseConstraintTorqueY=off  SenseConstraintTorqueZ=off  SenseTotalForce=off  SenseTotalForceX=off  SenseTotalForceY=off  SenseTotalForceZ=off  SenseTotalTorque=off  SenseTotalTorqueX=off  SenseTotalTorqueY=off  SenseTotalTorqueZ=off  CompositeWrenchDir=FollowerOnBase  CompositeWrenchFrame=BaseFrame  EquilibriumPosition=0  EquilibriumPositionUnits=rad  SpringStiffness=0  SpringStiffnessUnits=N*m/deg  DampingCoefficient=0  DampingCoefficientUnits=N*m/(deg/s)  TorqueActuationMode=ComputedTorque  MotionActuationMode=InputMotion  SensePosition=on  SenseVelocity=off  SenseAcceleration=off  SenseTorqueForce=off  SenseLowerLimitTorqueForce=off  SenseUpperLimitTorqueForce=off  LowerLimitSpecify=on  LowerLimitBound=robot_joints.q_limits(1)  LowerLimitBoundUnits=rad  LowerLimitStiffness=1e4  LowerLimitStiffnessUnits=N*m/deg  LowerLimitDamping=10  LowerLimitDampingUnits=N*m/(deg/s)  LowerLimitTransitionRegionWidth=0.1  LowerLimitTransitionRegionWidthUnits=deg  UpperLimitSpecify=on  UpperLimitBound=robot_joints.q_limits(2)  UpperLimitBoundUnits=rad  UpperLimitStiffness=1e4  UpperLimitStiffnessUnits=N*m/deg  UpperLimitDamping=10  UpperLimitDampingUnits=N*m/(deg/s)  UpperLimitTransitionRegionWidth=0.1  UpperLimitTransitionRegionWidthUnits=deg  PositionTargetSpecify=off  PositionTargetPriority=High  PositionTargetValue=0  PositionTargetValueUnits=deg  VelocityTargetSpecify=off  VelocityTargetPriority=High  VelocityTargetValue=0  VelocityTargetValueUnits=deg/s
  Simulink-PS Converter : nesl_utility/Simulink-PS Converter  PhysicalDomain=network_engine_domain  SubClassName=ps_input  LeftPortType=input  RightPortType=output  PseudoPeriodic=off  Frequencies=[]  NoiseDistribution=none  NoiseParameters=[]  Unit=1  AffineConversion=off  FilteringAndDerivatives=filter  SimscapeFilterOrder=2  InputFilterTimeConstant=0.001  UdotUserProvided=0
  Physical Art 1 : PMIOPort  Side=Right
  Physical Art 2 : PMIOPort  Port=2  Side=Right
  Servo Position (rad) : Outport
  wires:
  PWM Reference/1 -> LTI System/1
  LTI System/1 -> LTI System1/1
  LTI System1/1 -> DC to Rad/1(DC (0 -->1))  "DC after physical aproximation"
  Neutral Position (degrees)/1 -> Degrees to Radians/1
  DC to Rad/1(Position (rad)) -> Plus/1  "Position (rad)"
  Plus/1 -> Simulink-PS Converter/1  "Position (rad)"
  Degrees to Radians/1 -> Plus1/2, Plus/2
  PS-Simulink Converter/1 -> Plus1/1
  Plus1/1 -> Servo Position (rad)/1
  connections:
  PS-Simulink Converter/LConn1 -- Servomotor/RConn2
  Physical Art 2/RConn1 -- Servomotor/RConn1
  Servomotor/LConn1 -- Physical Art 1/RConn1
  Servomotor/LConn2 -- Simulink-PS Converter/RConn1

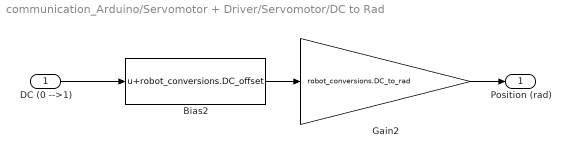
== system communication_Arduino/Servomotor + Driver/Servomotor/DC to Rad ==
  DC (0 -->1) : Inport
  Bias2 : Bias  Bias=robot_conversions.DC_offset  SaturateOnIntegerOverflow=off
  Gain2 : Gain  Gain=robot_conversions.DC_to_rad
  Position (rad) : Outport
  wires:
  DC (0 -->1)/1 -> Bias2/1
  Bias2/1 -> Gain2/1
  Gain2/1 -> Position (rad)/1

== system communication_Arduino/Servomotor + Driver 2/Servomotor/DC to Rad ==
  DC (0 -->1) : Inport
  Bias2 : Bias  Bias=robot_conversions.DC_offset  SaturateOnIntegerOverflow=off
  Gain2 : Gain  Gain=robot_conversions.DC_to_rad
  Position (rad) : Outport
  wires:
  DC (0 -->1)/1 -> Bias2/1
  Bias2/1 -> Gain2/1
  Gain2/1 -> Position (rad)/1

== system communication_Arduino/Servomotor + Driver 3/Servomotor/DC to Rad ==
  DC (0 -->1) : Inport
  Bias2 : Bias  Bias=robot_conversions.DC_offset  SaturateOnIntegerOverflow=off
  Gain2 : Gain  Gain=robot_conversions.DC_to_rad
  Position (rad) : Outport
  wires:
  DC (0 -->1)/1 -> Bias2/1
  Bias2/1 -> Gain2/1
  Gain2/1 -> Position (rad)/1
